simulink model "Experiment_cs"  (Simulink 8.8)
settings: Solver=ode5  StartTime=0.0  StopTime=inf  FixedStep=0.0005  RelTol=1e-3
PreLoadFcn:
  | check_NUTS_defined;
  | 
  | assignin('base',['model_closed_' bdroot],false);
InitFcn:
  | PreScanExperimentInitFcn(bdroot)
StopFcn:
  | PreScanExperimentStopFcn(bdroot)
undefined symbols (not defined in the file): DiscIntNeverNeededParam, FromPrescan, IdealSensors, psi, vd01, vd02, vd03, vd04, x, y
libraries: PreScanSimulinkLibrary x12, PreScanUsefulBlocks x8
(part 4 of 5)

== system Experiment_cs/Audi_A8_1/Dynamics_UserSpecified/SingleVehicle_01/Controller/CollectSensorData/PrescanProcess ==
  PrescanSimData : Inport
  Bus Creator : BusCreator  Inputs=12  OutDataTypeStr=Bus: PrescanSimData
      settings: InheritFromInputs=off
  SELF_Demux : Subsystem  Tag=DemuxSELF  mask(PreScan Demux Block:){}
      settings: DeleteFcn=PreScanBlockDeleteFcn;
      mask Display:
      | port_label('output',1,'x [m]')
      | port_label('output',2,'y [m]')
      | port_label('output',3,'z [m]','texmode','on')
      | port_label('output',4,'Rotx [deg]','texmode','on')
      | port_label('output',5,'Roty [deg]','texmode','on')
      | port_label('output',6,'Rotz [deg]','texmode','on')
      | port_label('output',7,'GPS lat [deg]','texmode','on')
      | port_label('output',8,'GPS long [deg]','texmode','on')
      | port_label('output',9,'GPS alt [m]','texmode','on')
      | port_label('output',10,'Velocity [m/s]')
      | port_label('output',11,'Heading [deg]')
      | port_label('output',12,'Yaw rate [deg/s]')
  PrescanSimDataBus : Outport
  wires:
  SELF_Demux/12(yaw rate [deg/s]) -> Bus Creator/12  "Yaw_rate"
  SELF_Demux/11(heading [deg]) -> Bus Creator/11  "heading"
  SELF_Demux/7(GPS lat [deg]) -> Bus Creator/7  "GPS_lat"
  SELF_Demux/6(rotz [deg]) -> Bus Creator/6  "Rotz"
  SELF_Demux/10(velocity [m/s]) -> Bus Creator/10  "u"
  SELF_Demux/8(GPS long [deg]) -> Bus Creator/8  "GPS_long"
  SELF_Demux/9(GPS alt [m]) -> Bus Creator/9  "GPS_alt"
  SELF_Demux/5(roty [deg]) -> Bus Creator/5  "Roty"
  SELF_Demux/4(rotx [deg]) -> Bus Creator/4  "Rotx"
  SELF_Demux/3(z [m]) -> Bus Creator/3  "z"
  SELF_Demux/2(y [m]) -> Bus Creator/2  "y"
  Bus Creator/1 -> PrescanSimDataBus/1
  PrescanSimData/1 -> SELF_Demux/1(SELF)
  SELF_Demux/1(x [m]) -> Bus Creator/1  "x"

== system Experiment_cs/Mazda_RX8_1/Dynamics_UserSpecified/SingleVehicle_01/Controller/CollectSensorData/IdealSensorsProcess ==
  VehicleState : Inport
  Bus Creator : BusCreator  Inputs=12  OutDataTypeStr=Bus: VehState
  Bus Selector : BusSelector  OutputSignals=x,y,z,theta,phi,psi,u,v,w,dtheta,dphi,dpsi
  IdealSensorsBus : Outport
  wires:
  Bus Creator/1 -> IdealSensorsBus/1
  Bus Selector/3 -> Bus Creator/3  "<z>"
  Bus Selector/12 -> Bus Creator/12  "<dpsi>"
  Bus Selector/5 -> Bus Creator/5  "<phi>"
  Bus Selector/2 -> Bus Creator/2  "<y>"
  Bus Selector/9 -> Bus Creator/9  "<w>"
  Bus Selector/4 -> Bus Creator/4  "<theta>"
  Bus Selector/6 -> Bus Creator/6  "<psi>"
  Bus Selector/11 -> Bus Creator/11  "<dphi>"
  Bus Selector/10 -> Bus Creator/10  "<dtheta>"
  Bus Selector/7 -> Bus Creator/7  "<u>"
  Bus Selector/8 -> Bus Creator/8  "<v>"
  Bus Selector/1 -> Bus Creator/1  "<x>"
  VehicleState/1 -> Bus Selector/1

== system Experiment_cs/Mazda_RX8_1/Dynamics_UserSpecified/SingleVehicle_01/Controller/CollectSensorData/PrescanProcess ==
  PrescanSimData : Inport
  Bus Creator : BusCreator  Inputs=12  OutDataTypeStr=Bus: PrescanSimData
      settings: InheritFromInputs=off
  SELF_Demux : Subsystem  Tag=DemuxSELF  mask(PreScan Demux Block:){}
      settings: DeleteFcn=PreScanBlockDeleteFcn;
      mask Display:
      | port_label('output',1,'x [m]')
      | port_label('output',2,'y [m]')
      | port_label('output',3,'z [m]','texmode','on')
      | port_label('output',4,'Rotx [deg]','texmode','on')
      | port_label('output',5,'Roty [deg]','texmode','on')
      | port_label('output',6,'Rotz [deg]','texmode','on')
      | port_label('output',7,'GPS lat [deg]','texmode','on')
      | port_label('output',8,'GPS long [deg]','texmode','on')
      | port_label('output',9,'GPS alt [m]','texmode','on')
      | port_label('output',10,'Velocity [m/s]')
      | port_label('output',11,'Heading [deg]')
      | port_label('output',12,'Yaw rate [deg/s]')
  PrescanSimDataBus : Outport
  wires:
  SELF_Demux/12(yaw rate [deg/s]) -> Bus Creator/12  "Yaw_rate"
  SELF_Demux/11(heading [deg]) -> Bus Creator/11  "heading"
  SELF_Demux/7(GPS lat [deg]) -> Bus Creator/7  "GPS_lat"
  SELF_Demux/6(rotz [deg]) -> Bus Creator/6  "Rotz"
  SELF_Demux/10(velocity [m/s]) -> Bus Creator/10  "u"
  SELF_Demux/8(GPS long [deg]) -> Bus Creator/8  "GPS_long"
  SELF_Demux/9(GPS alt [m]) -> Bus Creator/9  "GPS_alt"
  SELF_Demux/5(roty [deg]) -> Bus Creator/5  "Roty"
  SELF_Demux/4(rotx [deg]) -> Bus Creator/4  "Rotx"
  SELF_Demux/3(z [m]) -> Bus Creator/3  "z"
  SELF_Demux/2(y [m]) -> Bus Creator/2  "y"
  Bus Creator/1 -> PrescanSimDataBus/1
  PrescanSimData/1 -> SELF_Demux/1(SELF)
  SELF_Demux/1(x [m]) -> Bus Creator/1  "x"

== system Experiment_cs/Toyota_Yaris_1/Dynamics_UserSpecified/SingleVehicle_01/Controller/CollectSensorData/IdealSensorsProcess ==
  VehicleState : Inport
  Bus Creator : BusCreator  Inputs=12  OutDataTypeStr=Bus: VehState
  Bus Selector : BusSelector  OutputSignals=x,y,z,theta,phi,psi,u,v,w,dtheta,dphi,dpsi
  IdealSensorsBus : Outport
  wires:
  Bus Creator/1 -> IdealSensorsBus/1
  Bus Selector/3 -> Bus Creator/3  "<z>"
  Bus Selector/12 -> Bus Creator/12  "<dpsi>"
  Bus Selector/5 -> Bus Creator/5  "<phi>"
  Bus Selector/2 -> Bus Creator/2  "<y>"
  Bus Selector/9 -> Bus Creator/9  "<w>"
  Bus Selector/4 -> Bus Creator/4  "<theta>"
  Bus Selector/6 -> Bus Creator/6  "<psi>"
  Bus Selector/11 -> Bus Creator/11  "<dphi>"
  Bus Selector/10 -> Bus Creator/10  "<dtheta>"
  Bus Selector/7 -> Bus Creator/7  "<u>"
  Bus Selector/8 -> Bus Creator/8  "<v>"
  Bus Selector/1 -> Bus Creator/1  "<x>"
  VehicleState/1 -> Bus Selector/1

== system Experiment_cs/Toyota_Yaris_1/Dynamics_UserSpecified/SingleVehicle_01/Controller/CollectSensorData/PrescanProcess ==
  PrescanSimData : Inport
  Bus Creator : BusCreator  Inputs=12  OutDataTypeStr=Bus: PrescanSimData
      settings: InheritFromInputs=off
  SELF_Demux : Subsystem  Tag=DemuxSELF  mask(PreScan Demux Block:){}
      settings: DeleteFcn=PreScanBlockDeleteFcn;
      mask Display:
      | port_label('output',1,'x [m]')
      | port_label('output',2,'y [m]')
      | port_label('output',3,'z [m]','texmode','on')
      | port_label('output',4,'Rotx [deg]','texmode','on')
      | port_label('output',5,'Roty [deg]','texmode','on')
      | port_label('output',6,'Rotz [deg]','texmode','on')
      | port_label('output',7,'GPS lat [deg]','texmode','on')
      | port_label('output',8,'GPS long [deg]','texmode','on')
      | port_label('output',9,'GPS alt [m]','texmode','on')
      | port_label('output',10,'Velocity [m/s]')
      | port_label('output',11,'Heading [deg]')
      | port_label('output',12,'Yaw rate [deg/s]')
  PrescanSimDataBus : Outport
  wires:
  SELF_Demux/12(yaw rate [deg/s]) -> Bus Creator/12  "Yaw_rate"
  SELF_Demux/11(heading [deg]) -> Bus Creator/11  "heading"
  SELF_Demux/7(GPS lat [deg]) -> Bus Creator/7  "GPS_lat"
  SELF_Demux/6(rotz [deg]) -> Bus Creator/6  "Rotz"
  SELF_Demux/10(velocity [m/s]) -> Bus Creator/10  "u"
  SELF_Demux/8(GPS long [deg]) -> Bus Creator/8  "GPS_long"
  SELF_Demux/9(GPS alt [m]) -> Bus Creator/9  "GPS_alt"
  SELF_Demux/5(roty [deg]) -> Bus Creator/5  "Roty"
  SELF_Demux/4(rotx [deg]) -> Bus Creator/4  "Rotx"
  SELF_Demux/3(z [m]) -> Bus Creator/3  "z"
  SELF_Demux/2(y [m]) -> Bus Creator/2  "y"
  Bus Creator/1 -> PrescanSimDataBus/1
  PrescanSimData/1 -> SELF_Demux/1(SELF)
  SELF_Demux/1(x [m]) -> Bus Creator/1  "x"

== system Experiment_cs/Actros_2541_1/Dynamics_UserSpecified/SingleVehicle_01/Controller/CollectSensorData/PrescanProcess/SELF_Demux ==
  SELF : Inport
  Demux1 : Demux  Outputs=3
  Demux2 : Demux  Outputs=3
  Demux3 : Demux  Outputs=[3 3 1 1]
  Demux4 : Demux  Outputs=3
  Gain : Gain  Gain=180/pi
  Gain1 : Gain  Gain=180/pi
  Selector : Selector  InputPortWidth=3  IndexOptions=Index vector (dialog)  Indices=[3]  OutputSizes=1
  compas converter : Subsystem
  xyz2GPS : PreScanUsefulBlocks/xyz2GPS  CoordinateCount=1  GPS_base=[0.000000 0.000000 0.000]
  x [m] : Outport
  y [m] : Outport  Port=2
  z [m] : Outport  Port=3
  rotx [deg] : Outport  Port=4
  roty [deg] : Outport  Port=5
  rotz [deg] : Outport  Port=6
  GPS lat [deg] : Outport  Port=7
  GPS long [deg] : Outport  Port=8
  GPS alt [m] : Outport  Port=9
  velocity [m/s] : Outport  Port=10
  heading [deg] : Outport  Port=11
  yaw rate [deg/s] : Outport  Port=12
  wires:
  Selector/1 -> compas converter/1(rotz [rad])
  Gain/1 -> Demux2/1
  Demux1/1 -> x [m]/1
  Demux1/2 -> y [m]/1
  Demux1/3 -> z [m]/1
  Demux2/1 -> rotx [deg]/1
  Demux2/2 -> roty [deg]/1
  Demux2/3 -> rotz [deg]/1
  SELF/1 -> Demux3/1
  Demux3/1 -> Demux1/1, xyz2GPS/1
  Demux3/2 -> Selector/1, Gain/1
  Demux4/1 -> GPS lat [deg]/1
  Demux4/2 -> GPS long [deg]/1
  Demux4/3 -> GPS alt [m]/1
  xyz2GPS/1 -> Demux4/1
  compas converter/1(heading [deg]) -> heading [deg]/1
  Demux3/3 -> velocity [m/s]/1
  Gain1/1 -> yaw rate [deg/s]/1
  Demux3/4 -> Gain1/1

== system Experiment_cs/Audi_A8_1/Dynamics_UserSpecified/SingleVehicle_01/Controller/CollectSensorData/PrescanProcess/SELF_Demux ==
  SELF : Inport
  Demux1 : Demux  Outputs=3
  Demux2 : Demux  Outputs=3
  Demux3 : Demux  Outputs=[3 3 1 1]
  Demux4 : Demux  Outputs=3
  Gain : Gain  Gain=180/pi
  Gain1 : Gain  Gain=180/pi
  Selector : Selector  InputPortWidth=3  IndexOptions=Index vector (dialog)  Indices=[3]  OutputSizes=1
  compas converter : Subsystem
  xyz2GPS : PreScanUsefulBlocks/xyz2GPS  CoordinateCount=1  GPS_base=[0.000000 0.000000 0.000]
  x [m] : Outport
  y [m] : Outport  Port=2
  z [m] : Outport  Port=3
  rotx [deg] : Outport  Port=4
  roty [deg] : Outport  Port=5
  rotz [deg] : Outport  Port=6
  GPS lat [deg] : Outport  Port=7
  GPS long [deg] : Outport  Port=8
  GPS alt [m] : Outport  Port=9
  velocity [m/s] : Outport  Port=10
  heading [deg] : Outport  Port=11
  yaw rate [deg/s] : Outport  Port=12
  wires:
  Selector/1 -> compas converter/1(rotz [rad])
  Gain/1 -> Demux2/1
  Demux1/1 -> x [m]/1
  Demux1/2 -> y [m]/1
  Demux1/3 -> z [m]/1
  Demux2/1 -> rotx [deg]/1
  Demux2/2 -> roty [deg]/1
  Demux2/3 -> rotz [deg]/1
  SELF/1 -> Demux3/1
  Demux3/1 -> Demux1/1, xyz2GPS/1
  Demux3/2 -> Selector/1, Gain/1
  Demux4/1 -> GPS lat [deg]/1
  Demux4/2 -> GPS long [deg]/1
  Demux4/3 -> GPS alt [m]/1
  xyz2GPS/1 -> Demux4/1
  compas converter/1(heading [deg]) -> heading [deg]/1
  Demux3/3 -> velocity [m/s]/1
  Gain1/1 -> yaw rate [deg/s]/1
  Demux3/4 -> Gain1/1

== system Experiment_cs/Mazda_RX8_1/Dynamics_UserSpecified/SingleVehicle_01/Controller/CollectSensorData/PrescanProcess/SELF_Demux ==
  SELF : Inport
  Demux1 : Demux  Outputs=3
  Demux2 : Demux  Outputs=3
  Demux3 : Demux  Outputs=[3 3 1 1]
  Demux4 : Demux  Outputs=3
  Gain : Gain  Gain=180/pi
  Gain1 : Gain  Gain=180/pi
  Selector : Selector  InputPortWidth=3  IndexOptions=Index vector (dialog)  Indices=[3]  OutputSizes=1
  compas converter : Subsystem
  xyz2GPS : PreScanUsefulBlocks/xyz2GPS  CoordinateCount=1  GPS_base=[0.000000 0.000000 0.000]
  x [m] : Outport
  y [m] : Outport  Port=2
  z [m] : Outport  Port=3
  rotx [deg] : Outport  Port=4
  roty [deg] : Outport  Port=5
  rotz [deg] : Outport  Port=6
  GPS lat [deg] : Outport  Port=7
  GPS long [deg] : Outport  Port=8
  GPS alt [m] : Outport  Port=9
  velocity [m/s] : Outport  Port=10
  heading [deg] : Outport  Port=11
  yaw rate [deg/s] : Outport  Port=12
  wires:
  Selector/1 -> compas converter/1(rotz [rad])
  Gain/1 -> Demux2/1
  Demux1/1 -> x [m]/1
  Demux1/2 -> y [m]/1
  Demux1/3 -> z [m]/1
  Demux2/1 -> rotx [deg]/1
  Demux2/2 -> roty [deg]/1
  Demux2/3 -> rotz [deg]/1
  SELF/1 -> Demux3/1
  Demux3/1 -> Demux1/1, xyz2GPS/1
  Demux3/2 -> Selector/1, Gain/1
  Demux4/1 -> GPS lat [deg]/1
  Demux4/2 -> GPS long [deg]/1
  Demux4/3 -> GPS alt [m]/1
  xyz2GPS/1 -> Demux4/1
  compas converter/1(heading [deg]) -> heading [deg]/1
  Demux3/3 -> velocity [m/s]/1
  Gain1/1 -> yaw rate [deg/s]/1
  Demux3/4 -> Gain1/1

== system Experiment_cs/Toyota_Yaris_1/Dynamics_UserSpecified/SingleVehicle_01/Controller/CollectSensorData/PrescanProcess/SELF_Demux ==
  SELF : Inport
  Demux1 : Demux  Outputs=3
  Demux2 : Demux  Outputs=3
  Demux3 : Demux  Outputs=[3 3 1 1]
  Demux4 : Demux  Outputs=3
  Gain : Gain  Gain=180/pi
  Gain1 : Gain  Gain=180/pi
  Selector : Selector  InputPortWidth=3  IndexOptions=Index vector (dialog)  Indices=[3]  OutputSizes=1
  compas converter : Subsystem
  xyz2GPS : PreScanUsefulBlocks/xyz2GPS  CoordinateCount=1  GPS_base=[0.000000 0.000000 0.000]
  x [m] : Outport
  y [m] : Outport  Port=2
  z [m] : Outport  Port=3
  rotx [deg] : Outport  Port=4
  roty [deg] : Outport  Port=5
  rotz [deg] : Outport  Port=6
  GPS lat [deg] : Outport  Port=7
  GPS long [deg] : Outport  Port=8
  GPS alt [m] : Outport  Port=9
  velocity [m/s] : Outport  Port=10
  heading [deg] : Outport  Port=11
  yaw rate [deg/s] : Outport  Port=12
  wires:
  Selector/1 -> compas converter/1(rotz [rad])
  Gain/1 -> Demux2/1
  Demux1/1 -> x [m]/1
  Demux1/2 -> y [m]/1
  Demux1/3 -> z [m]/1
  Demux2/1 -> rotx [deg]/1
  Demux2/2 -> roty [deg]/1
  Demux2/3 -> rotz [deg]/1
  SELF/1 -> Demux3/1
  Demux3/1 -> Demux1/1, xyz2GPS/1
  Demux3/2 -> Selector/1, Gain/1
  Demux4/1 -> GPS lat [deg]/1
  Demux4/2 -> GPS long [deg]/1
  Demux4/3 -> GPS alt [m]/1
  xyz2GPS/1 -> Demux4/1
  compas converter/1(heading [deg]) -> heading [deg]/1
  Demux3/3 -> velocity [m/s]/1
  Gain1/1 -> yaw rate [deg/s]/1
  Demux3/4 -> Gain1/1

== system Experiment_cs/Actros_2541_1/Dynamics_UserSpecified/SingleVehicle_01/Controller/CollectSensorData/PrescanProcess/SELF_Demux/compas converter ==
  rotz [rad] : Inport
  cart2compas : Subsystem
  rad2deg : Gain  Gain=180/pi
  heading [deg] : Outport
  wires:
  rad2deg/1 -> cart2compas/1(Angle [deg])
  rotz [rad]/1 -> rad2deg/1
  cart2compas/1(heading [deg]) -> heading [deg]/1

== system Experiment_cs/Audi_A8_1/Dynamics_UserSpecified/SingleVehicle_01/Controller/CollectSensorData/PrescanProcess/SELF_Demux/compas converter ==
  rotz [rad] : Inport
  cart2compas : Subsystem
  rad2deg : Gain  Gain=180/pi
  heading [deg] : Outport
  wires:
  rad2deg/1 -> cart2compas/1(Angle [deg])
  rotz [rad]/1 -> rad2deg/1
  cart2compas/1(heading [deg]) -> heading [deg]/1

== system Experiment_cs/Mazda_RX8_1/Dynamics_UserSpecified/SingleVehicle_01/Controller/CollectSensorData/PrescanProcess/SELF_Demux/compas converter ==
  rotz [rad] : Inport
  cart2compas : Subsystem
  rad2deg : Gain  Gain=180/pi
  heading [deg] : Outport
  wires:
  rad2deg/1 -> cart2compas/1(Angle [deg])
  rotz [rad]/1 -> rad2deg/1
  cart2compas/1(heading [deg]) -> heading [deg]/1

== system Experiment_cs/Toyota_Yaris_1/Dynamics_UserSpecified/SingleVehicle_01/Controller/CollectSensorData/PrescanProcess/SELF_Demux/compas converter ==
  rotz [rad] : Inport
  cart2compas : Subsystem
  rad2deg : Gain  Gain=180/pi
  heading [deg] : Outport
  wires:
  rad2deg/1 -> cart2compas/1(Angle [deg])
  rotz [rad]/1 -> rad2deg/1
  cart2compas/1(heading [deg]) -> heading [deg]/1

== system Experiment_cs/Actros_2541_1/Dynamics_UserSpecified/SingleVehicle_01/Controller/CollectSensorData/PrescanProcess/SELF_Demux/compas converter/cart2compas ==
  Angle [deg] : Inport
  Constant : Constant  Value=90
  Constant1 : Constant  Value=360
  Gain : Gain  Gain=1/360
  Gain1 : Gain  Gain=360
  Gain2 : Gain  Gain=-1
  Rounding Function : Rounding
  Sum : Sum  Inputs=|-+
  Sum1 : Sum  Inputs=-+|
  Sum2 : Sum  Inputs=++|
  heading [deg] : Outport
  wires:
  Gain/1 -> Rounding Function/1
  Rounding Function/1 -> Gain1/1
  Gain1/1 -> Sum/1
  Angle [deg]/1 -> Sum1/2
  Sum/1 -> Gain2/1
  Sum1/1 -> Gain/1, Sum/2
  Constant/1 -> Sum1/1
  Gain2/1 -> Sum2/2
  Constant1/1 -> Sum2/1
  Sum2/1 -> heading [deg]/1

== system Experiment_cs/Audi_A8_1/Dynamics_UserSpecified/SingleVehicle_01/Controller/CollectSensorData/PrescanProcess/SELF_Demux/compas converter/cart2compas ==
  Angle [deg] : Inport
  Constant : Constant  Value=90
  Constant1 : Constant  Value=360
  Gain : Gain  Gain=1/360
  Gain1 : Gain  Gain=360
  Gain2 : Gain  Gain=-1
  Rounding Function : Rounding
  Sum : Sum  Inputs=|-+
  Sum1 : Sum  Inputs=-+|
  Sum2 : Sum  Inputs=++|
  heading [deg] : Outport
  wires:
  Gain/1 -> Rounding Function/1
  Rounding Function/1 -> Gain1/1
  Gain1/1 -> Sum/1
  Angle [deg]/1 -> Sum1/2
  Sum/1 -> Gain2/1
  Sum1/1 -> Gain/1, Sum/2
  Constant/1 -> Sum1/1
  Gain2/1 -> Sum2/2
  Constant1/1 -> Sum2/1
  Sum2/1 -> heading [deg]/1

== system Experiment_cs/Mazda_RX8_1/Dynamics_UserSpecified/SingleVehicle_01/Controller/CollectSensorData/PrescanProcess/SELF_Demux/compas converter/cart2compas ==
  Angle [deg] : Inport
  Constant : Constant  Value=90
  Constant1 : Constant  Value=360
  Gain : Gain  Gain=1/360
  Gain1 : Gain  Gain=360
  Gain2 : Gain  Gain=-1
  Rounding Function : Rounding
  Sum : Sum  Inputs=|-+
  Sum1 : Sum  Inputs=-+|
  Sum2 : Sum  Inputs=++|
  heading [deg] : Outport
  wires:
  Gain/1 -> Rounding Function/1
  Rounding Function/1 -> Gain1/1
  Gain1/1 -> Sum/1
  Angle [deg]/1 -> Sum1/2
  Sum/1 -> Gain2/1
  Sum1/1 -> Gain/1, Sum/2
  Constant/1 -> Sum1/1
  Gain2/1 -> Sum2/2
  Constant1/1 -> Sum2/1
  Sum2/1 -> heading [deg]/1

== system Experiment_cs/Toyota_Yaris_1/Dynamics_UserSpecified/SingleVehicle_01/Controller/CollectSensorData/PrescanProcess/SELF_Demux/compas converter/cart2compas ==
  Angle [deg] : Inport
  Constant : Constant  Value=90
  Constant1 : Constant  Value=360
  Gain : Gain  Gain=1/360
  Gain1 : Gain  Gain=360
  Gain2 : Gain  Gain=-1
  Rounding Function : Rounding
  Sum : Sum  Inputs=|-+
  Sum1 : Sum  Inputs=-+|
  Sum2 : Sum  Inputs=++|
  heading [deg] : Outport
  wires:
  Gain/1 -> Rounding Function/1
  Rounding Function/1 -> Gain1/1
  Gain1/1 -> Sum/1
  Angle [deg]/1 -> Sum1/2
  Sum/1 -> Gain2/1
  Sum1/1 -> Gain/1, Sum/2
  Constant/1 -> Sum1/1
  Gain2/1 -> Sum2/2
  Constant1/1 -> Sum2/1
  Sum2/1 -> heading [deg]/1

== matlab function Audi_A8_1/Dynamics_UserSpecified/SingleVehicle_01/Controller/CtlMainBusUnitDelayAndInit/MATLAB Function ==
  data: u input double; y output Bus: ControllerMainBus; veh_struct parameter double
function y = DelayAndInitCtlBus(u, veh_struct)
coder.extrinsic('exist')
persistent a

y0 = struct;

y0.ActuationCmdBus = struct;
y0.ActuationCmdBus.steering_cmd = 0;
y0.ActuationCmdBus.decel_cmd = 0;
y0.ActuationCmdBus.accel_cmd = 0;

y0.ArbitratedActuationReq = struct;
y0.ArbitratedActuationReq.v_des = 0;
y0.ArbitratedActuationReq.a_des = 0;
y0.ArbitratedActuationReq.psi_des = 0;
y0.ArbitratedActuationReq.dpsi_des = 0;


y0.FunctionFeatures = struct;
y0.FunctionFeatures.wpFollower = struct;
y0.FunctionFeatures.wpFollower.v_des = 0;
y0.FunctionFeatures.wpFollower.a_des = 0;
y0.FunctionFeatures.wpFollower.psi_des = 0;
y0.FunctionFeatures.wpFollower.dpsi_des = 0;


y0.situationBus = struct;
y0.situationBus.wP = struct;

y0.situationBus.wP.finalWayPoint = struct;
y0.situationBus.wP.finalWayPoint.x = 0;
y0.situationBus.wP.finalWayPoint.y = 0;
y0.situationBus.wP.finalWayPoint.z = 0;
y0.situationBus.wP.finalWayPoint.treach = 0;

y0.situationBus.wP.currentWayPoint = struct;
y0.situationBus.wP.currentWayPoint.x = 0;
y0.situationBus.wP.currentWayPoint.y = 0;
y0.situationBus.wP.currentWayPoint.z = 0;
y0.situationBus.wP.currentWayPoint.treach = 0;

y0.situationBus.wP.finalWayPointIndex = uint16(1);
y0.situationBus.wP.currentWayPointIndex = uint16(10);

%y0.situationBus.wP.wayPointArray = struct;
wPArray = struct;
wPArray.x = 0;
wPArray.y = 0;
wPArray.z = 0;
wPArray.treach = 0;
y0.situationBus.wP.wayPointArray = repmat(wPArray,100,1);


y0.situationBus.selfAwarenessBus = struct;
y0.situationBus.selfAwarenessBus.x = 0;
y0.situationBus.selfAwarenessBus.y = 0;
y0.situationBus.selfAwarenessBus.z = 0;
y0.situationBus.selfAwarenessBus.theta = 0;
y0.situationBus.selfAwarenessBus.phi = 0;
y0.situationBus.selfAwarenessBus.psi = 0;
y0.situationBus.selfAwarenessBus.u = 0;
y0.situationBus.selfAwarenessBus.v = 0;
y0.situationBus.selfAwarenessBus.w = 0;
y0.situationBus.selfAwarenessBus.dtheta = 0;
y0.situationBus.selfAwarenessBus.dphi = 0;
y0.situationBus.selfAwarenessBus.dpsi = 0;
y0.IdealSensors = struct;
y0.IdealSensors.x = 0;
y0.IdealSensors.y = 0;
y0.IdealSensors.z = 0;
y0.IdealSensors.theta = 0;
y0.IdealSensors.phi = 0;
y0.IdealSensors.psi = 0;
y0.IdealSensors.u = 0;
y0.IdealSensors.v = 0;
y0.IdealSensors.w = 0;
y0.IdealSensors.dtheta = 0;
y0.IdealSensors.dphi = 0;
y0.IdealSensors.dpsi = 0;
y0.FromPrescan = struct;
y0.FromPrescan.x = 0;
y0.FromPrescan.y = 0;
y0.FromPrescan.z = 0;
y0.FromPrescan.Rotx = 0;
y0.FromPrescan.Roty = 0;
y0.FromPrescan.Rotz = 0;
y0.FromPrescan.GPS_lat = 0;
y0.FromPrescan.GPS_long = 0;
y0.FromPrescan.u = 0;
y0.FromPrescan.GPS_alt = 0;
y0.FromPrescan.heading = 0;
y0.FromPrescan.Yaw_rate = 0;



if isempty(a)
    a = 1;
    y = y0;
    y.situationBus.wP.wayPointArray = veh_struct.initialWayPointsArray;
    y.situationBus.wP.currentWayPointIndex = veh_struct.initialCurrentWayPointIndex;
    y.situationBus.wP.finalWayPointIndex = veh_struct.initialFinalWayPointIndex;

else
    y = u;
end

== matlab function Audi_A8_1/Dynamics_UserSpecified/SingleVehicle_01/VehStateBusUnitDelayAndInit/MATLAB Function ==
  data: u input double; y output Bus: VehState
function y = DelayAndInitVehState(u)
persistent a
y0 = struct;
y0.x = 1;
y0.y = 2;
y0.z = 0;
y0.theta = 0;
y0.phi = 0;
y0.psi = 0;
y0.u = 0;
y0.v = 0;
y0.w = 0;
y0.dtheta = 0;
y0.dphi = 0;
y0.dpsi = 0;

%y0 = VehState_MATLABStruct;
if isempty(a)
    a = 1;
    y = y0;
else
    y = u;
end

== matlab function Audi_A8_1/Dynamics_UserSpecified/SingleVehicle_01/Controller/SituationalAwareness/situationAwareness ==
  data: prevSituation input Bus: situationBus; newSituation output Bus: situationBus; prescanSimData input Bus: PrescanSimData; idealSensors input Bus: VehState; veh_struct parameter double
function newSituation = calcSituationAwareness(prevSituation,prescanSimData,idealSensors, veh_struct)

newSituation = prevSituation;


newSituation.selfAwarenessBus.x = idealSensors.x;
newSituation.selfAwarenessBus.y = idealSensors.y;
newSituation.selfAwarenessBus.z = idealSensors.z;
newSituation.selfAwarenessBus.theta = idealSensors.theta;
newSituation.selfAwarenessBus.phi = idealSensors.phi;
newSituation.selfAwarenessBus.psi = idealSensors.psi;
newSituation.selfAwarenessBus.u = idealSensors.u;
newSituation.selfAwarenessBus.v = idealSensors.v;
newSituation.selfAwarenessBus.w = idealSensors.w;
newSituation.selfAwarenessBus.dtheta = idealSensors.dtheta;
newSituation.selfAwarenessBus.dphi = idealSensors.dphi;
newSituation.selfAwarenessBus.dpsi = idealSensors.dpsi;


end

== matlab function Audi_A8_1/Dynamics_UserSpecified/SingleVehicle_01/Controller/FeaturedFunctions/wpFollower ==
  data: prevWpAction input Bus: wpFollower; prevSituation input Bus: situationBus; wpAction output Bus: wpFollower; veh_struct parameter double; newSituation output Bus: situationBus
function [wpAction, newSituation] = wpFollower(prevWpAction, prevSituation, veh_struct)

currentIndex = prevSituation.wP.currentWayPointIndex;
if currentIndex < 1
    currentIndex = uint16(1);
end
finalIndex = prevSituation.wP.finalWayPointIndex;

xd = prevSituation.wP.wayPointArray(currentIndex).x;
yd = prevSituation.wP.wayPointArray(currentIndex).y;
xa = prevSituation.selfAwarenessBus.x;
ya = prevSituation.selfAwarenessBus.y;
howClose = norm([xd-xa, yd-ya]);

if howClose < veh_struct.wpControl.wayPointThreshold
    if (currentIndex == finalIndex)
        currentIndex = uint16(1);
    else
        currentIndex = uint16(currentIndex + 1);
    end
end

newSituation = prevSituation;
newSituation.wP.currentWayPointIndex = uint16(currentIndex);
newSituation.wP.currentWayPoint.x = newSituation.wP.wayPointArray(currentIndex).x;
newSituation.wP.currentWayPoint.y = newSituation.wP.wayPointArray(currentIndex).y;
newSituation.wP.currentWayPoint.z = newSituation.wP.wayPointArray(currentIndex).z;
newSituation.wP.currentWayPoint.treach = newSituation.wP.wayPointArray(currentIndex).treach;

v_des_raw = min(veh_struct.wpControl.v_des_max, howClose / veh_struct.wpControl.howClose_saturate * veh_struct.wpControl.v_des_max);
psi_des_raw = atan2((yd-ya),(xd-xa));

% if psi_des_raw < 0
%     
%     dbg = 1;
%     
% end
    

v_des_old = prevWpAction.v_des;
psi_des_old = prevWpAction.psi_des;

a_des = veh_struct.wpControl.v_des_filter.lambda * (v_des_raw - v_des_old);
v_des = v_des_old + veh_struct.CONTROL_OS_SAMPLETIME * a_des;

dpsi_des = veh_struct.wpControl.psi_des_filter.lambda * (psi_des_raw - psi_des_old);
psi_des = psi_des_old + veh_struct.CONTROL_OS_SAMPLETIME * dpsi_des;
% psi_des = mod(psi_des, 2 * pi);


wpAction.v_des = v_des;
wpAction.a_des = a_des;
wpAction.psi_des = psi_des;
wpAction.dpsi_des = dpsi_des;

end

== matlab function Audi_A8_1/Dynamics_UserSpecified/SingleVehicle_01/Controller/StrategicArbitration/Arbitration ==
  data: FunctionFeatures input Bus: FunctionFeatures; ArbitratedReq output Bus: ArbitratedActuationReq
function ArbitratedReq = Arbitrate(FunctionFeatures)

ArbitratedReq.v_des = FunctionFeatures.wpFollower.v_des;
ArbitratedReq.a_des = FunctionFeatures.wpFollower.a_des;
ArbitratedReq.psi_des = FunctionFeatures.wpFollower.psi_des;
ArbitratedReq.dpsi_des = FunctionFeatures.wpFollower.dpsi_des;

end

== matlab function Audi_A8_1/Dynamics_UserSpecified/SingleVehicle_01/Controller/Actuation/DynamicControls ==
  data: ActReq input Bus: ArbitratedActuationReq; Ctl input Bus: ControllerMainBus; ActCmds output Bus: ActuationCmdBus; ActCmdsPrev input Bus: ActuationCmdBus
function ActCmds  = fcn(ActReq, Ctl, ActCmdsPrev)

v_des = ActReq.v_des;
a_des = ActReq.a_des;
psi_des = ActReq.psi_des;
dpsi_des = ActReq.dpsi_des;

% ActCmds = ActCmdsPrev;
% ActCmds.accel_cmd = 0;
% ActCmds.decel_cmd = 0;
% ActCmds.steering_cmd = 0.1;

ActCmds = ActCmdsPrev;

if a_des >= 0
    ActCmds.accel_cmd = ActReq.a_des;
    ActCmds.decel_cmd = 0;
else
    ActCmds.accel_cmd = 0;
    ActCmds.decel_cmd = ActReq.a_des;
end

psi_des = unwrap(psi_des);
Ctl.IdealSensors.psi = unwrap(Ctl.IdealSensors.psi);

ActCmds.steering_cmd = 3.5*(psi_des - Ctl.IdealSensors.psi);

== matlab function Audi_A8_1/Dynamics_UserSpecified/SingleVehicle_01/VehicleDynamics/KinematicVehicleModel ==
  data: u input double; delta input double; dX output double; psi input double; dY output double; dpsi output double; veh_struct parameter double
function [dX,dY,dpsi] = fcn(u,delta, psi, veh_struct)

lf = veh_struct.lf;
lr = veh_struct.lr;

% psi = unwrap(psi);
% delta = unwrap(delta);

beta = atan( lr /(lf + lr) * tan(delta));

% beta = unwrap(beta);

dX = u * cos(psi + beta);
dY = u * sin(psi + beta);
dpsi = u / lr * sin(beta);

== matlab function Audi_A8_1/Dynamics_UserSpecified/SingleVehicle_01/Controller/Actuation/ActuatorDrivers ==
  data: ActCmds input Bus: ActuationCmdBus; accel_cmd output double; decel_cmd output double; steering_cmd output double
function [accel_cmd, decel_cmd, steering_cmd]  = fcn(ActCmds)

accel_cmd = ActCmds.accel_cmd;
decel_cmd = ActCmds.decel_cmd;
steering_cmd = ActCmds.steering_cmd;

end

== matlab function Actros_2541_1/Dynamics_UserSpecified/SingleVehicle_01/Controller/Actuation/ActuatorDrivers ==
  data: ActCmds input Bus: ActuationCmdBus; accel_cmd output double; decel_cmd output double; steering_cmd output double
function [accel_cmd, decel_cmd, steering_cmd]  = fcn(ActCmds)

accel_cmd = ActCmds.accel_cmd;
decel_cmd = ActCmds.decel_cmd;
steering_cmd = ActCmds.steering_cmd;

end

== matlab function Actros_2541_1/Dynamics_UserSpecified/SingleVehicle_01/Controller/Actuation/DynamicControls ==
  data: ActReq input Bus: ArbitratedActuationReq; Ctl input Bus: ControllerMainBus; ActCmds output Bus: ActuationCmdBus; ActCmdsPrev input Bus: ActuationCmdBus
function ActCmds  = fcn(ActReq, Ctl, ActCmdsPrev)

v_des = ActReq.v_des;
a_des = ActReq.a_des;
psi_des = ActReq.psi_des;
dpsi_des = ActReq.dpsi_des;

% ActCmds = ActCmdsPrev;
% ActCmds.accel_cmd = 0;
% ActCmds.decel_cmd = 0;
% ActCmds.steering_cmd = 0.1;

ActCmds = ActCmdsPrev;

if a_des >= 0
    ActCmds.accel_cmd = ActReq.a_des;
    ActCmds.decel_cmd = 0;
else
    ActCmds.accel_cmd = 0;
    ActCmds.decel_cmd = ActReq.a_des;
end

psi_des = unwrap(psi_des);
Ctl.IdealSensors.psi = unwrap(Ctl.IdealSensors.psi);

ActCmds.steering_cmd = 3.5*(psi_des - Ctl.IdealSensors.psi);

== matlab function Actros_2541_1/Dynamics_UserSpecified/SingleVehicle_01/Controller/CtlMainBusUnitDelayAndInit/MATLAB Function ==
  data: u input double; y output Bus: ControllerMainBus; veh_struct parameter double
function y = DelayAndInitCtlBus(u, veh_struct)
coder.extrinsic('exist')
persistent a

y0 = struct;

y0.ActuationCmdBus = struct;
y0.ActuationCmdBus.steering_cmd = 0;
y0.ActuationCmdBus.decel_cmd = 0;
y0.ActuationCmdBus.accel_cmd = 0;

y0.ArbitratedActuationReq = struct;
y0.ArbitratedActuationReq.v_des = 0;
y0.ArbitratedActuationReq.a_des = 0;
y0.ArbitratedActuationReq.psi_des = 0;
y0.ArbitratedActuationReq.dpsi_des = 0;


y0.FunctionFeatures = struct;
y0.FunctionFeatures.wpFollower = struct;
y0.FunctionFeatures.wpFollower.v_des = 0;
y0.FunctionFeatures.wpFollower.a_des = 0;
y0.FunctionFeatures.wpFollower.psi_des = 0;
y0.FunctionFeatures.wpFollower.dpsi_des = 0;


y0.situationBus = struct;
y0.situationBus.wP = struct;

y0.situationBus.wP.finalWayPoint = struct;
y0.situationBus.wP.finalWayPoint.x = 0;
y0.situationBus.wP.finalWayPoint.y = 0;
y0.situationBus.wP.finalWayPoint.z = 0;
y0.situationBus.wP.finalWayPoint.treach = 0;

y0.situationBus.wP.currentWayPoint = struct;
y0.situationBus.wP.currentWayPoint.x = 0;
y0.situationBus.wP.currentWayPoint.y = 0;
y0.situationBus.wP.currentWayPoint.z = 0;
y0.situationBus.wP.currentWayPoint.treach = 0;

y0.situationBus.wP.finalWayPointIndex = uint16(1);
y0.situationBus.wP.currentWayPointIndex = uint16(10);

%y0.situationBus.wP.wayPointArray = struct;
wPArray = struct;
wPArray.x = 0;
wPArray.y = 0;
wPArray.z = 0;
wPArray.treach = 0;
y0.situationBus.wP.wayPointArray = repmat(wPArray,100,1);


y0.situationBus.selfAwarenessBus = struct;
y0.situationBus.selfAwarenessBus.x = 0;
y0.situationBus.selfAwarenessBus.y = 0;
y0.situationBus.selfAwarenessBus.z = 0;
y0.situationBus.selfAwarenessBus.theta = 0;
y0.situationBus.selfAwarenessBus.phi = 0;
y0.situationBus.selfAwarenessBus.psi = 0;
y0.situationBus.selfAwarenessBus.u = 0;
y0.situationBus.selfAwarenessBus.v = 0;
y0.situationBus.selfAwarenessBus.w = 0;
y0.situationBus.selfAwarenessBus.dtheta = 0;
y0.situationBus.selfAwarenessBus.dphi = 0;
y0.situationBus.selfAwarenessBus.dpsi = 0;
y0.IdealSensors = struct;
y0.IdealSensors.x = 0;
y0.IdealSensors.y = 0;
y0.IdealSensors.z = 0;
y0.IdealSensors.theta = 0;
y0.IdealSensors.phi = 0;
y0.IdealSensors.psi = 0;
y0.IdealSensors.u = 0;
y0.IdealSensors.v = 0;
y0.IdealSensors.w = 0;
y0.IdealSensors.dtheta = 0;
y0.IdealSensors.dphi = 0;
y0.IdealSensors.dpsi = 0;
y0.FromPrescan = struct;
y0.FromPrescan.x = 0;
y0.FromPrescan.y = 0;
y0.FromPrescan.z = 0;
y0.FromPrescan.Rotx = 0;
y0.FromPrescan.Roty = 0;
y0.FromPrescan.Rotz = 0;
y0.FromPrescan.GPS_lat = 0;
y0.FromPrescan.GPS_long = 0;
y0.FromPrescan.u = 0;
y0.FromPrescan.GPS_alt = 0;
y0.FromPrescan.heading = 0;
y0.FromPrescan.Yaw_rate = 0;



if isempty(a)
    a = 1;
    y = y0;
    y.situationBus.wP.wayPointArray = veh_struct.initialWayPointsArray;
    y.situationBus.wP.currentWayPointIndex = veh_struct.initialCurrentWayPointIndex;
    y.situationBus.wP.finalWayPointIndex = veh_struct.initialFinalWayPointIndex;

else
    y = u;
end

== matlab function Actros_2541_1/Dynamics_UserSpecified/SingleVehicle_01/Controller/FeaturedFunctions/wpFollower ==
  data: prevWpAction input Bus: wpFollower; prevSituation input Bus: situationBus; wpAction output Bus: wpFollower; veh_struct parameter double; newSituation output Bus: situationBus
function [wpAction, newSituation] = wpFollower(prevWpAction, prevSituation, veh_struct)

currentIndex = prevSituation.wP.currentWayPointIndex;
if currentIndex < 1
    currentIndex = uint16(1);
end
finalIndex = prevSituation.wP.finalWayPointIndex;

xd = prevSituation.wP.wayPointArray(currentIndex).x;
yd = prevSituation.wP.wayPointArray(currentIndex).y;
xa = prevSituation.selfAwarenessBus.x;
ya = prevSituation.selfAwarenessBus.y;
howClose = norm([xd-xa, yd-ya]);

if howClose < veh_struct.wpControl.wayPointThreshold
    if (currentIndex == finalIndex)
        currentIndex = uint16(1);
    else
        currentIndex = uint16(currentIndex + 1);
    end
end

newSituation = prevSituation;
newSituation.wP.currentWayPointIndex = uint16(currentIndex);
newSituation.wP.currentWayPoint.x = newSituation.wP.wayPointArray(currentIndex).x;
newSituation.wP.currentWayPoint.y = newSituation.wP.wayPointArray(currentIndex).y;
newSituation.wP.currentWayPoint.z = newSituation.wP.wayPointArray(currentIndex).z;
newSituation.wP.currentWayPoint.treach = newSituation.wP.wayPointArray(currentIndex).treach;

v_des_raw = min(veh_struct.wpControl.v_des_max, howClose / veh_struct.wpControl.howClose_saturate * veh_struct.wpControl.v_des_max);
psi_des_raw = atan2((yd-ya),(xd-xa));

% if psi_des_raw < 0
%     
%     dbg = 1;
%     
% end
    

v_des_old = prevWpAction.v_des;
psi_des_old = prevWpAction.psi_des;

a_des = veh_struct.wpControl.v_des_filter.lambda * (v_des_raw - v_des_old);
v_des = v_des_old + veh_struct.CONTROL_OS_SAMPLETIME * a_des;

dpsi_des = veh_struct.wpControl.psi_des_filter.lambda * (psi_des_raw - psi_des_old);
psi_des = psi_des_old + veh_struct.CONTROL_OS_SAMPLETIME * dpsi_des;
% psi_des = mod(psi_des, 2 * pi);


wpAction.v_des = v_des;
wpAction.a_des = a_des;
wpAction.psi_des = psi_des;
wpAction.dpsi_des = dpsi_des;

end

== matlab function Actros_2541_1/Dynamics_UserSpecified/SingleVehicle_01/Controller/SituationalAwareness/situationAwareness ==
  data: prevSituation input Bus: situationBus; newSituation output Bus: situationBus; prescanSimData input Bus: PrescanSimData; idealSensors input Bus: VehState; veh_struct parameter double
function newSituation = calcSituationAwareness(prevSituation,prescanSimData,idealSensors, veh_struct)

newSituation = prevSituation;


newSituation.selfAwarenessBus.x = idealSensors.x;
newSituation.selfAwarenessBus.y = idealSensors.y;
newSituation.selfAwarenessBus.z = idealSensors.z;
newSituation.selfAwarenessBus.theta = idealSensors.theta;
newSituation.selfAwarenessBus.phi = idealSensors.phi;
newSituation.selfAwarenessBus.psi = idealSensors.psi;
newSituation.selfAwarenessBus.u = idealSensors.u;
newSituation.selfAwarenessBus.v = idealSensors.v;
newSituation.selfAwarenessBus.w = idealSensors.w;
newSituation.selfAwarenessBus.dtheta = idealSensors.dtheta;
newSituation.selfAwarenessBus.dphi = idealSensors.dphi;
newSituation.selfAwarenessBus.dpsi = idealSensors.dpsi;


end

== matlab function Actros_2541_1/Dynamics_UserSpecified/SingleVehicle_01/Controller/StrategicArbitration/Arbitration ==
  data: FunctionFeatures input Bus: FunctionFeatures; ArbitratedReq output Bus: ArbitratedActuationReq
function ArbitratedReq = Arbitrate(FunctionFeatures)

ArbitratedReq.v_des = FunctionFeatures.wpFollower.v_des;
ArbitratedReq.a_des = FunctionFeatures.wpFollower.a_des;
ArbitratedReq.psi_des = FunctionFeatures.wpFollower.psi_des;
ArbitratedReq.dpsi_des = FunctionFeatures.wpFollower.dpsi_des;

end

== matlab function Actros_2541_1/Dynamics_UserSpecified/SingleVehicle_01/VehStateBusUnitDelayAndInit/MATLAB Function ==
  data: u input double; y output Bus: VehState
function y = DelayAndInitVehState(u)
persistent a
y0 = struct;
y0.x = 1;
y0.y = 2;
y0.z = 0;
y0.theta = 0;
y0.phi = 0;
y0.psi = 0;
y0.u = 0;
y0.v = 0;
y0.w = 0;
y0.dtheta = 0;
y0.dphi = 0;
y0.dpsi = 0;

%y0 = VehState_MATLABStruct;
if isempty(a)
    a = 1;
    y = y0;
else
    y = u;
end

== matlab function Actros_2541_1/Dynamics_UserSpecified/SingleVehicle_01/VehicleDynamics/KinematicVehicleModel ==
  data: u input double; delta input double; dX output double; psi input double; dY output double; dpsi output double; veh_struct parameter double
function [dX,dY,dpsi] = fcn(u,delta, psi, veh_struct)

lf = veh_struct.lf;
lr = veh_struct.lr;

% psi = unwrap(psi);
% delta = unwrap(delta);

beta = atan( lr /(lf + lr) * tan(delta));

% beta = unwrap(beta);

dX = u * cos(psi + beta);
dY = u * sin(psi + beta);
dpsi = u / lr * sin(beta);

== matlab function Mazda_RX8_1/Dynamics_UserSpecified/SingleVehicle_01/Controller/Actuation/ActuatorDrivers ==
  data: ActCmds input Bus: ActuationCmdBus; accel_cmd output double; decel_cmd output double; steering_cmd output double
function [accel_cmd, decel_cmd, steering_cmd]  = fcn(ActCmds)

accel_cmd = ActCmds.accel_cmd;
decel_cmd = ActCmds.decel_cmd;
steering_cmd = ActCmds.steering_cmd;

end

== matlab function Mazda_RX8_1/Dynamics_UserSpecified/SingleVehicle_01/Controller/Actuation/DynamicControls ==
  data: ActReq input Bus: ArbitratedActuationReq; Ctl input Bus: ControllerMainBus; ActCmds output Bus: ActuationCmdBus; ActCmdsPrev input Bus: ActuationCmdBus
function ActCmds  = fcn(ActReq, Ctl, ActCmdsPrev)

v_des = ActReq.v_des;
a_des = ActReq.a_des;
psi_des = ActReq.psi_des;
dpsi_des = ActReq.dpsi_des;

% ActCmds = ActCmdsPrev;
% ActCmds.accel_cmd = 0;
% ActCmds.decel_cmd = 0;
% ActCmds.steering_cmd = 0.1;

ActCmds = ActCmdsPrev;

if a_des >= 0
    ActCmds.accel_cmd = ActReq.a_des;
    ActCmds.decel_cmd = 0;
else
    ActCmds.accel_cmd = 0;
    ActCmds.decel_cmd = ActReq.a_des;
end

psi_des = unwrap(psi_des);
Ctl.IdealSensors.psi = unwrap(Ctl.IdealSensors.psi);

ActCmds.steering_cmd = 3.5*(psi_des - Ctl.IdealSensors.psi);

== matlab function Mazda_RX8_1/Dynamics_UserSpecified/SingleVehicle_01/Controller/CtlMainBusUnitDelayAndInit/MATLAB Function ==
  data: u input double; y output Bus: ControllerMainBus; veh_struct parameter double
function y = DelayAndInitCtlBus(u, veh_struct)
coder.extrinsic('exist')
persistent a

y0 = struct;

y0.ActuationCmdBus = struct;
y0.ActuationCmdBus.steering_cmd = 0;
y0.ActuationCmdBus.decel_cmd = 0;
y0.ActuationCmdBus.accel_cmd = 0;

y0.ArbitratedActuationReq = struct;
y0.ArbitratedActuationReq.v_des = 0;
y0.ArbitratedActuationReq.a_des = 0;
y0.ArbitratedActuationReq.psi_des = 0;
y0.ArbitratedActuationReq.dpsi_des = 0;


y0.FunctionFeatures = struct;
y0.FunctionFeatures.wpFollower = struct;
y0.FunctionFeatures.wpFollower.v_des = 0;
y0.FunctionFeatures.wpFollower.a_des = 0;
y0.FunctionFeatures.wpFollower.psi_des = 0;
y0.FunctionFeatures.wpFollower.dpsi_des = 0;


y0.situationBus = struct;
y0.situationBus.wP = struct;

y0.situationBus.wP.finalWayPoint = struct;
y0.situationBus.wP.finalWayPoint.x = 0;
y0.situationBus.wP.finalWayPoint.y = 0;
y0.situationBus.wP.finalWayPoint.z = 0;
y0.situationBus.wP.finalWayPoint.treach = 0;

y0.situationBus.wP.currentWayPoint = struct;
y0.situationBus.wP.currentWayPoint.x = 0;
y0.situationBus.wP.currentWayPoint.y = 0;
y0.situationBus.wP.currentWayPoint.z = 0;
y0.situationBus.wP.currentWayPoint.treach = 0;

y0.situationBus.wP.finalWayPointIndex = uint16(1);
y0.situationBus.wP.currentWayPointIndex = uint16(10);

%y0.situationBus.wP.wayPointArray = struct;
wPArray = struct;
wPArray.x = 0;
wPArray.y = 0;
wPArray.z = 0;
wPArray.treach = 0;
y0.situationBus.wP.wayPointArray = repmat(wPArray,100,1);


y0.situationBus.selfAwarenessBus = struct;
y0.situationBus.selfAwarenessBus.x = 0;
y0.situationBus.selfAwarenessBus.y = 0;
y0.situationBus.selfAwarenessBus.z = 0;
y0.situationBus.selfAwarenessBus.theta = 0;
y0.situationBus.selfAwarenessBus.phi = 0;
y0.situationBus.selfAwarenessBus.psi = 0;
y0.situationBus.selfAwarenessBus.u = 0;
y0.situationBus.selfAwarenessBus.v = 0;
y0.situationBus.selfAwarenessBus.w = 0;
y0.situationBus.selfAwarenessBus.dtheta = 0;
y0.situationBus.selfAwarenessBus.dphi = 0;
y0.situationBus.selfAwarenessBus.dpsi = 0;
y0.IdealSensors = struct;
y0.IdealSensors.x = 0;
y0.IdealSensors.y = 0;
y0.IdealSensors.z = 0;
y0.IdealSensors.theta = 0;
y0.IdealSensors.phi = 0;
y0.IdealSensors.psi = 0;
y0.IdealSensors.u = 0;
y0.IdealSensors.v = 0;
y0.IdealSensors.w = 0;
y0.IdealSensors.dtheta = 0;
y0.IdealSensors.dphi = 0;
y0.IdealSensors.dpsi = 0;
y0.FromPrescan = struct;
y0.FromPrescan.x = 0;
y0.FromPrescan.y = 0;
y0.FromPrescan.z = 0;
y0.FromPrescan.Rotx = 0;
y0.FromPrescan.Roty = 0;
y0.FromPrescan.Rotz = 0;
y0.FromPrescan.GPS_lat = 0;
y0.FromPrescan.GPS_long = 0;
y0.FromPrescan.u = 0;
y0.FromPrescan.GPS_alt = 0;
y0.FromPrescan.heading = 0;
y0.FromPrescan.Yaw_rate = 0;



if isempty(a)
    a = 1;
    y = y0;
    y.situationBus.wP.wayPointArray = veh_struct.initialWayPointsArray;
    y.situationBus.wP.currentWayPointIndex = veh_struct.initialCurrentWayPointIndex;
    y.situationBus.wP.finalWayPointIndex = veh_struct.initialFinalWayPointIndex;

else
    y = u;
end

== matlab function Mazda_RX8_1/Dynamics_UserSpecified/SingleVehicle_01/Controller/FeaturedFunctions/wpFollower ==
  data: prevWpAction input Bus: wpFollower; prevSituation input Bus: situationBus; wpAction output Bus: wpFollower; veh_struct parameter double; newSituation output Bus: situationBus
function [wpAction, newSituation] = wpFollower(prevWpAction, prevSituation, veh_struct)

currentIndex = prevSituation.wP.currentWayPointIndex;
if currentIndex < 1
    currentIndex = uint16(1);
end
finalIndex = prevSituation.wP.finalWayPointIndex;

xd = prevSituation.wP.wayPointArray(currentIndex).x;
yd = prevSituation.wP.wayPointArray(currentIndex).y;
xa = prevSituation.selfAwarenessBus.x;
ya = prevSituation.selfAwarenessBus.y;
howClose = norm([xd-xa, yd-ya]);

if howClose < veh_struct.wpControl.wayPointThreshold
    if (currentIndex == finalIndex)
        currentIndex = uint16(1);
    else
        currentIndex = uint16(currentIndex + 1);
    end
end

newSituation = prevSituation;
newSituation.wP.currentWayPointIndex = uint16(currentIndex);
newSituation.wP.currentWayPoint.x = newSituation.wP.wayPointArray(currentIndex).x;
newSituation.wP.currentWayPoint.y = newSituation.wP.wayPointArray(currentIndex).y;
newSituation.wP.currentWayPoint.z = newSituation.wP.wayPointArray(currentIndex).z;
newSituation.wP.currentWayPoint.treach = newSituation.wP.wayPointArray(currentIndex).treach;

v_des_raw = min(veh_struct.wpControl.v_des_max, howClose / veh_struct.wpControl.howClose_saturate * veh_struct.wpControl.v_des_max);
psi_des_raw = atan2((yd-ya),(xd-xa));

% if psi_des_raw < 0
%     
%     dbg = 1;
%     
% end
    

v_des_old = prevWpAction.v_des;
psi_des_old = prevWpAction.psi_des;

a_des = veh_struct.wpControl.v_des_filter.lambda * (v_des_raw - v_des_old);
v_des = v_des_old + veh_struct.CONTROL_OS_SAMPLETIME * a_des;

dpsi_des = veh_struct.wpControl.psi_des_filter.lambda * (psi_des_raw - psi_des_old);
psi_des = psi_des_old + veh_struct.CONTROL_OS_SAMPLETIME * dpsi_des;
% psi_des = mod(psi_des, 2 * pi);


wpAction.v_des = v_des;
wpAction.a_des = a_des;
wpAction.psi_des = psi_des;
wpAction.dpsi_des = dpsi_des;

end

== matlab function Mazda_RX8_1/Dynamics_UserSpecified/SingleVehicle_01/Controller/SituationalAwareness/situationAwareness ==
  data: prevSituation input Bus: situationBus; newSituation output Bus: situationBus; prescanSimData input Bus: PrescanSimData; idealSensors input Bus: VehState; veh_struct parameter double
function newSituation = calcSituationAwareness(prevSituation,prescanSimData,idealSensors, veh_struct)

newSituation = prevSituation;


newSituation.selfAwarenessBus.x = idealSensors.x;
newSituation.selfAwarenessBus.y = idealSensors.y;
newSituation.selfAwarenessBus.z = idealSensors.z;
newSituation.selfAwarenessBus.theta = idealSensors.theta;
newSituation.selfAwarenessBus.phi = idealSensors.phi;
newSituation.selfAwarenessBus.psi = idealSensors.psi;
newSituation.selfAwarenessBus.u = idealSensors.u;
newSituation.selfAwarenessBus.v = idealSensors.v;
newSituation.selfAwarenessBus.w = idealSensors.w;
newSituation.selfAwarenessBus.dtheta = idealSensors.dtheta;
newSituation.selfAwarenessBus.dphi = idealSensors.dphi;
newSituation.selfAwarenessBus.dpsi = idealSensors.dpsi;


end

== matlab function Mazda_RX8_1/Dynamics_UserSpecified/SingleVehicle_01/Controller/StrategicArbitration/Arbitration ==
  data: FunctionFeatures input Bus: FunctionFeatures; ArbitratedReq output Bus: ArbitratedActuationReq
function ArbitratedReq = Arbitrate(FunctionFeatures)

ArbitratedReq.v_des = FunctionFeatures.wpFollower.v_des;
ArbitratedReq.a_des = FunctionFeatures.wpFollower.a_des;
ArbitratedReq.psi_des = FunctionFeatures.wpFollower.psi_des;
ArbitratedReq.dpsi_des = FunctionFeatures.wpFollower.dpsi_des;

end

== matlab function Mazda_RX8_1/Dynamics_UserSpecified/SingleVehicle_01/VehStateBusUnitDelayAndInit/MATLAB Function ==
  data: u input double; y output Bus: VehState
function y = DelayAndInitVehState(u)
persistent a
y0 = struct;
y0.x = 1;
y0.y = 2;
y0.z = 0;
y0.theta = 0;
y0.phi = 0;
y0.psi = 0;
y0.u = 0;
y0.v = 0;
y0.w = 0;
y0.dtheta = 0;
y0.dphi = 0;
y0.dpsi = 0;

%y0 = VehState_MATLABStruct;
if isempty(a)
    a = 1;
    y = y0;
else
    y = u;
end

== matlab function Mazda_RX8_1/Dynamics_UserSpecified/SingleVehicle_01/VehicleDynamics/KinematicVehicleModel ==
  data: u input double; delta input double; dX output double; psi input double; dY output double; dpsi output double; veh_struct parameter double
function [dX,dY,dpsi] = fcn(u,delta, psi, veh_struct)

lf = veh_struct.lf;
lr = veh_struct.lr;

% psi = unwrap(psi);
% delta = unwrap(delta);

beta = atan( lr /(lf + lr) * tan(delta));

% beta = unwrap(beta);

dX = u * cos(psi + beta);
dY = u * sin(psi + beta);
dpsi = u / lr * sin(beta);

== matlab function Toyota_Yaris_1/Dynamics_UserSpecified/SingleVehicle_01/Controller/Actuation/ActuatorDrivers ==
  data: ActCmds input Bus: ActuationCmdBus; accel_cmd output double; decel_cmd output double; steering_cmd output double
function [accel_cmd, decel_cmd, steering_cmd]  = fcn(ActCmds)

accel_cmd = ActCmds.accel_cmd;
decel_cmd = ActCmds.decel_cmd;
steering_cmd = ActCmds.steering_cmd;

end

== matlab function Toyota_Yaris_1/Dynamics_UserSpecified/SingleVehicle_01/Controller/Actuation/DynamicControls ==
  data: ActReq input Bus: ArbitratedActuationReq; Ctl input Bus: ControllerMainBus; ActCmds output Bus: ActuationCmdBus; ActCmdsPrev input Bus: ActuationCmdBus
function ActCmds  = fcn(ActReq, Ctl, ActCmdsPrev)

v_des = ActReq.v_des;
a_des = ActReq.a_des;
psi_des = ActReq.psi_des;
dpsi_des = ActReq.dpsi_des;

% ActCmds = ActCmdsPrev;
% ActCmds.accel_cmd = 0;
% ActCmds.decel_cmd = 0;
% ActCmds.steering_cmd = 0.1;

ActCmds = ActCmdsPrev;

if a_des >= 0
    ActCmds.accel_cmd = ActReq.a_des;
    ActCmds.decel_cmd = 0;
else
    ActCmds.accel_cmd = 0;
    ActCmds.decel_cmd = ActReq.a_des;
end

psi_des = unwrap(psi_des);
Ctl.IdealSensors.psi = unwrap(Ctl.IdealSensors.psi);

ActCmds.steering_cmd = 3.5*(psi_des - Ctl.IdealSensors.psi);
